simulink model "TPractica1"  (R2024a)
settings: Solver=VariableStepAuto  StartTime=0.0  StopTime=25.0  RelTol=1e-3
undefined symbols (not defined in the file): g, l1, l2, m1, m2, magnitude
settings Model: Creator=52331  LastModifiedBy=52331

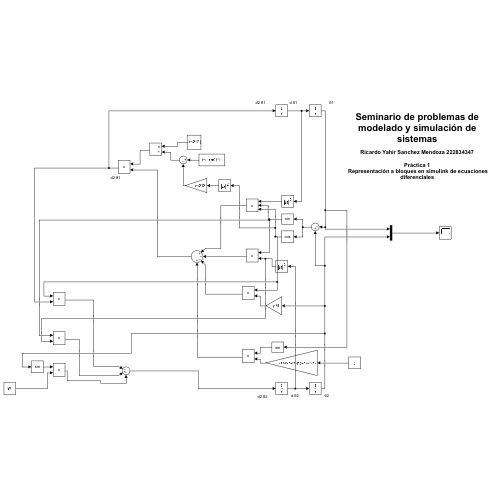
[thumbnail: Simulink's stored preview of the top-level diagram]
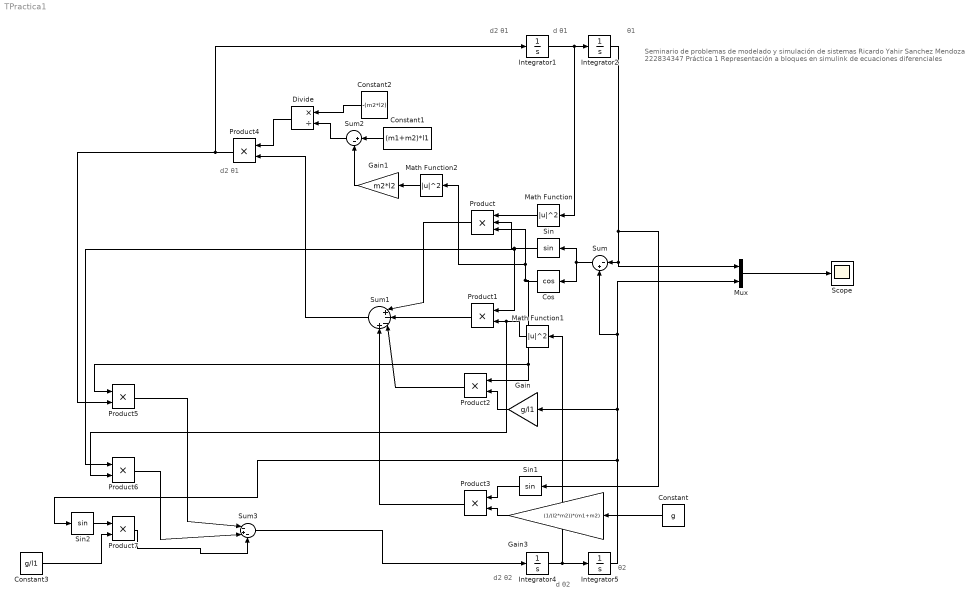
== system TPractica1 ==
  note: Seminario de problemas de modelado y simulación de sistemas
      |
      | Ricardo Yahir Sanchez Mendoza 222834347
      |
      | Práctica 1
      | Representación a bloques en simulink de ecuaciones diferenciales
  note: d2 θ1
  note: d θ1
  note: θ1
  note: d θ2
  note: θ2
  note: d2 θ2
  note: d2 θ1
  Constant : Constant  Value=g
  Constant1 : Constant  Value=(m1+m2)*l1
  Constant2 : Constant  Value=-(m2*l2)
  Constant3 : Constant  Value=g/l1
  Cos : Trigonometry  Operator=cos
  Divide : Product  Inputs=*/
  Gain : Gain  Gain=g/l1
  Gain1 : Gain  Gain=m2*l2
  Gain3 : Gain  Gain=(1/(l2*m2))*(m1+m2)
  Integrator1 : Integrator
  Integrator2 : Integrator
  Integrator4 : Integrator
  Integrator5 : Integrator  InitialCondition=deg2rad(35)
  Math Function : Math  Operator=magnitude^2
  Math Function1 : Math  Operator=magnitude^2
  Math Function2 : Math  Operator=magnitude^2
  Mux : Mux  Inputs=2
  Product : Product  Inputs=3
  Product{1..7} (7 alike) : Product
  Scope : Scope
  Sin : Trigonometry
  Sin1 : Trigonometry
  Sin2 : Trigonometry
  Sum : Sum  Inputs=|-+
  Sum1 : Sum  Inputs=|+--+
  Sum2 : Sum  Inputs=|+-
  Sum3 : Sum  Inputs=|-+-
  wires:
  Integrator1/1 -> Math Function/1, Integrator2/1
  Integrator4/1 -> Integrator5/1, Math Function1/1
  Math Function/1 -> Product/1
  Sin/1 -> Product6/1, Product1/1, Product/2
  Cos/1 -> Product/3, Math Function2/1, Product5/1, Product2/1
  Integrator2/1 -> Mux/1, Sum/1, Sin1/1
  Sum/1 -> Cos/1, Sin/1
  Math Function1/1 -> Product6/2, Product1/2
  Gain/1 -> Product2/2
  Constant/1 -> Gain3/1
  Sin1/1 -> Product3/1
  Gain3/1 -> Product3/2
  Product/1 -> Sum1/1
  Product1/1 -> Sum1/2
  Product2/1 -> Sum1/3
  Product3/1 -> Sum1/4
  Constant1/1 -> Sum2/1
  Math Function2/1 -> Gain1/1
  Gain1/1 -> Sum2/2
  Sum2/1 -> Divide/2
  Constant2/1 -> Divide/1
  Sum1/1 -> Product4/2
  Divide/1 -> Product4/1
  Product4/1 -> Product5/2, Integrator1/1
  Sin2/1 -> Product7/1
  Integrator5/1 -> Mux/2, Sum/2, Gain/1, Sin2/1
  Constant3/1 -> Product7/2
  Product5/1 -> Sum3/1
  Product6/1 -> Sum3/2
  Product7/1 -> Sum3/3
  Sum3/1 -> Integrator4/1
  Mux/1 -> Scope/1
